simulink model "fm2"  (R2013a)
settings: Solver=FixedStepDiscrete  StartTime=0.0  StopTime=180  RelTol=1e-3
undefined symbols (not defined in the file): dfilt, get
libraries: dsparch4 x5, commsynccomp2 x2, dspsigops x2, dspxfrm3 x1, simulink x1, commdigbbndpm3 x1, commsink2 x1, commtimrec2 x1, rtlsdr x1
settings Model: Creator=tomas  LastModifiedBy=tomas

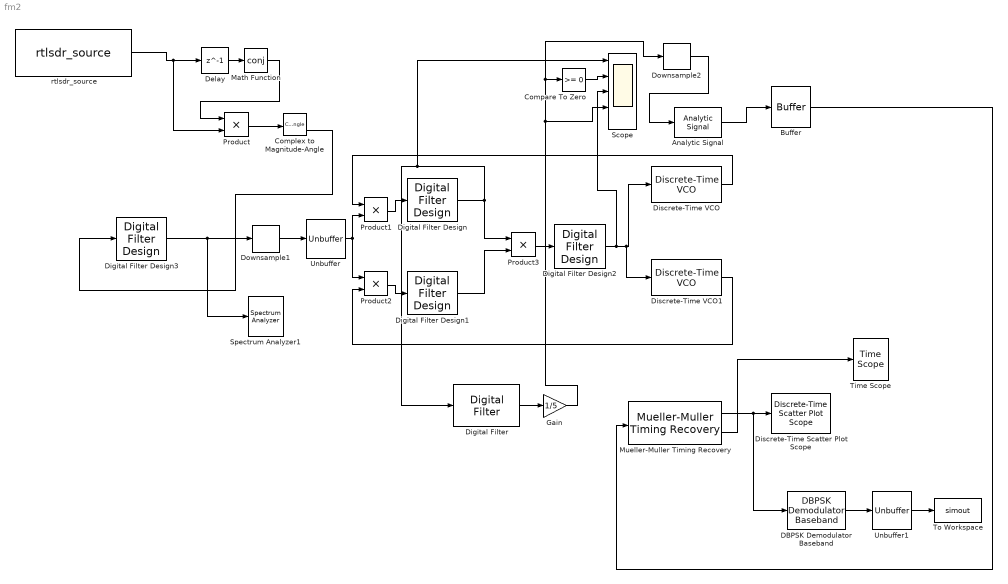
== system fm2 ==
  Analytic Signal : dspxfrm3/Analytic Signal  N=100  InputProcessing=Columns as channels (frame based)
  Buffer : Buffer  N=15  TreatMby1Signals=One channel
  Compare To Zero : simulink/Logic and Bit Operations/Compare To Zero  relop=>=  OutDataTypeStr=boolean
  Complex to Magnitude-Angle : ComplexToMagnitudeAngle
  DBPSK Demodulator Baseband : commdigbbndpm3/DBPSK Demodulator Baseband  Ph=0  outDtype=Inherit via internal rule
  Delay : Delay  DelayLength=1  InputProcessing=Columns as channels (frame based)
  Digital Filter Design{,1..3} (4 alike) : dsparch4/Digital Filter Design  mwdsp_browser_bugfix_var=off
  Digital Filter : dsparch4/Digital Filter  TypePopup=FIR (all zeros)  IIRFiltStruct=Direct form II transposed  AllPoleFiltStruct=Direct form  FIRFiltStruct=Direct form  CoeffSource=Specify via dialog  NumCoeffs=[sin((2*pi*1187.5/(250000/14))*[-7.5:1:7.5])]  DenCoeffs=[1 0.1]  BiQuadCoeffs=[1 0.3 0.4 1 0.1 0.2]  LatticeCoeffs=[0.2 0.4]  denIgnore=on  FiltPerSampPopup=One filter per frame  IC=0  ICnum=0  ICden=0  roundingMode=Floor  overflowMode=off  ScaleValues=1  scaleValueFracLength=14  stageInFracLength=15  stageOutFracLength=15  FilterSource=Specify via dialog  dfiltObjectName=dfilt.dffir([1 2 1])  InputProcessing=Columns as channels (frame based)
  Discrete-Time Scatter Plot Scope : commsink2/Discrete-Time Scatter Plot Scope  Tag=ScatterPlot  sampPerSymb=1  offsetEye=0  numTraces=200  numNewFrames=200  LineMarkers=.  LineColors=b  fading=on  render=on  AxisGrid=on  xMin=-3.3  xMax=3.315  yMin=-3.3  yMax=3.315  inphaseLabel=In-phase Amplitude  quadratureLabel=Quadrature Amplitude  openScopeAtSimStart=on  FrameNumber=off  FigPos=get(0,'defaultfigureposition');  figTitle=Scatter Plot  numLinesMax=8  block_type_=scatter
  Discrete-Time VCO : commsynccomp2/Discrete-Time VCO  Ac=10  Fc=3428.6  Kc=1e2  Ph=0  ts=-1
  Discrete-Time VCO1 : commsynccomp2/Discrete-Time VCO  Ac=10  Fc=3428.6  Kc=1e2  Ph=pi/2  ts=-1
  Downsample1 : dspsigops/Downsample  N=14  phase=0  InputProcessing=Columns as channels (frame based)  RateOptions=Enforce single-rate processing  smode=Allow multirate  fmode=Maintain input frame size  ic=0
  Downsample2 : dspsigops/Downsample  N=1  phase=0  InputProcessing=Columns as channels (frame based)  RateOptions=Allow multirate processing  smode=Allow multirate  fmode=Maintain input frame size  ic=0
  Gain : Gain  Gain=1/5
  Math Function : Math  Operator=conj  SaturateOnIntegerOverflow=on
  Mueller-Muller Timing Recovery : commtimrec2/Mueller-Muller Timing Recovery  sampPerSymbol=15  propGain=0.05  resetMode=None
  Product{,1..3} (4 alike) : Product
  Scope : Scope  NumInputPorts=5
      settings: YMin=-2~0~-0.25~-2~-1  YMax=2.5~1~0.1~2~1  MaxDataPoints=1500000
  Spectrum Analyzer1 : SpectrumAnalyzer
      settings: CopyFcn=scopeextensions.ScopeBlock.callback(gcbh, 'onBlockCopy', gcbh);  DeleteFcn=scopeextensions.ScopeBlock.callback(gcbh, 'onBlockDelete');  PreSaveFcn=scopeextensions.ScopeBlock.callback(gcbh, 'onModelSave');  NameChangeFcn=scopeextensions.ScopeBlock.callback(gcbh, 'onBlockRename');  CloseFcn=scopeextensions.ScopeBlock.callback(gcbh, 'onBlockClose');  PreDeleteFcn=scopeextensions.ScopeBlock.callback(gcbh, 'onBlockPreDelete');
  Time Scope : TimeScope  DefaultConfigurationName=spbscopes.TimeScopeBlockCfg
      settings: CopyFcn=scopeextensions.ScopeBlock.callback(gcbh, 'onBlockCopy', gcbh);  DeleteFcn=scopeextensions.ScopeBlock.callback(gcbh, 'onBlockDelete');  PreSaveFcn=scopeextensions.ScopeBlock.callback(gcbh, 'onModelSave');  NameChangeFcn=scopeextensions.ScopeBlock.callback(gcbh, 'onBlockRename');  CloseFcn=scopeextensions.ScopeBlock.callback(gcbh, 'onBlockClose');  PreDeleteFcn=scopeextensions.ScopeBlock.callback(gcbh, 'onBlockPreDelete');
  To Workspace : ToWorkspace  VariableName=simout  SampleTime=-1  SaveFormat=Timeseries
  Unbuffer : Unbuffer  SampleBasedProcessing=Same as frame based
  Unbuffer1 : Unbuffer  SampleBasedProcessing=Same as frame based
  rtlsdr_source : rtlsdr/rtlsdr_source  rtlsdr_device_index=0  rtlsdr_query=off  rtlsdr_samplerate=250000  rtlsdr_frame_length=1050  rtlsdr_frame_type=Frame  rtlsdr_frequency=88.8e6  rtlsdr_frequency_tune=off  rtlsdr_gain=0  rtlsdr_gain_tune=off  rtlsdr_agc_on=on  rtlsdr_restore_block=off
  wires:
  Digital Filter Design2/1 -> Scope/3, Discrete-Time VCO1/1, Discrete-Time VCO/1
  Discrete-Time VCO/1 -> Product1/1
  Discrete-Time VCO1/1 -> Product2/2
  Digital Filter Design1/1 -> Product3/2
  Product3/1 -> Digital Filter Design2/1
  Product2/1 -> Digital Filter Design1/1
  Product1/1 -> Digital Filter Design/1
  Compare To Zero/1 -> Scope/2
  Delay/1 -> Math Function/1
  Math Function/1 -> Product/1
  Product/1 -> Complex to Magnitude-Angle/1
  Unbuffer/1 -> Product2/1, Product1/2
  Downsample1/1 -> Unbuffer/1
  Complex to Magnitude-Angle/2 -> Digital Filter Design3/1
  Digital Filter Design3/1 -> Spectrum Analyzer1/1, Downsample1/1
  rtlsdr_source/1 -> Product/2, Delay/1
  Digital Filter Design/1 -> Product3/1, Digital Filter/1, Scope/1
  Downsample2/1 -> Analytic Signal/1
  Digital Filter/1 -> Gain/1
  Gain/1 -> Downsample2/1, Compare To Zero/1, Scope/4
  Analytic Signal/1 -> Buffer/1
  Buffer/1 -> Mueller-Muller Timing Recovery/1
  Mueller-Muller Timing Recovery/1 -> DBPSK Demodulator Baseband/1, Discrete-Time Scatter Plot Scope/1
  DBPSK Demodulator Baseband/1 -> Unbuffer1/1
  Unbuffer1/1 -> To Workspace/1
  Mueller-Muller Timing Recovery/2 -> Time Scope/1
